simulink model "styremodell"  (R2023b)
settings: Solver=VariableStepAuto  StartTime=0.0  StopTime=30  RelTol=1e-3
undefined symbols (not defined in the file): areal_front, areal_side, areal_topp, bidrag_gir_front, bidrag_gir_side, bidrag_rull_side, bidrag_rull_topp, bidrag_stamp_front, bidrag_stamp_topp, Cd_front, Cd_side, Cd_topp, Fb, g, masse, r_Fb, r_motor_gir, r_motor_rull, r_motor_stamp, tetthet_vann, theta_motor_gir, theta_motor_rull, theta_motor_stamp, treghetsmoment_gir, treghetsmoment_rull, treghetsmoment_stamp
libraries: simulink_extras x8
settings Model: Creator=kristianbirkeland  LastModifiedBy=bmm1
settings DebuggingCC: UnconnectedInputMsg=warning  UnconnectedOutputMsg=warning  UnconnectedLineMsg=warning
settings ModelReferenceCC: EnableRefExpFcnMdlSchedulingChecks=on
settings RTWCC: DLArmComputeVersion=19.05

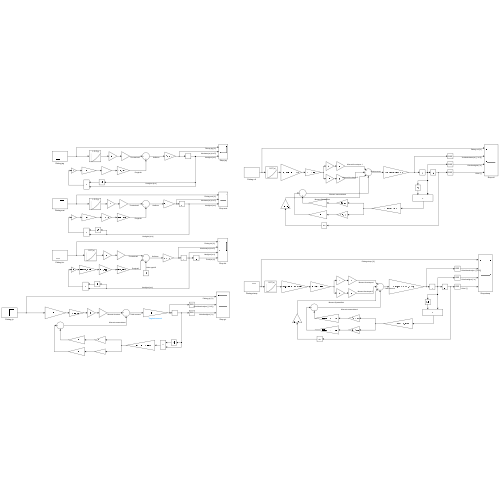
[thumbnail: Simulink's stored preview of the top-level diagram]
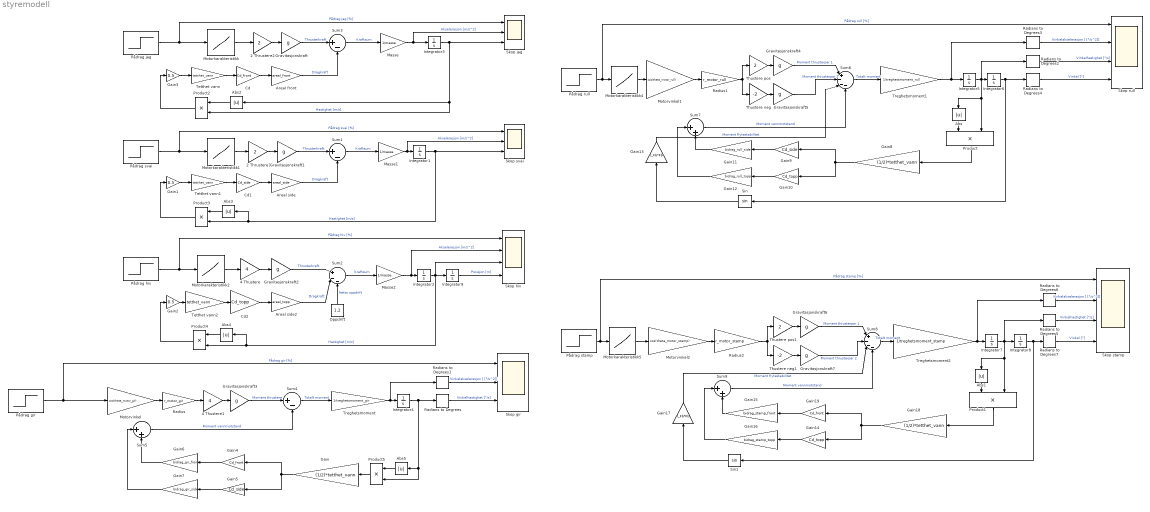
== system styremodell ==
  2 Thrustere1 : Gain  Gain=2
  2 Thrustere2 : Gain  Gain=2
  4 Thustere : Gain  Gain=4
  4 Thustere1 : Gain  Gain=4
  Abs{,1..5} (6 alike) : Abs  SaturateOnIntegerOverflow=off
  Areal front : Gain  Gain=areal_front
  Areal side : Gain  Gain=areal_side
  Areal side2 : Gain  Gain=areal_topp
  Cd : Gain  Gain=Cd_front
  Cd1 : Gain  Gain=Cd_side
  Cd2 : Gain  Gain=Cd_topp
  Gain : Gain  Gain=(1/2)*tetthet_vann
  Gain1 : Gain  Gain=0.5
  Gain10 : Gain  Gain=Cd_topp
  Gain11 : Gain  Gain=bidrag_rull_side
  Gain12 : Gain  Gain=bidrag_rull_topp
  Gain13 : Gain  Gain=r_Fb*Fb
  Gain14 : Gain  Gain=Cd_topp
  Gain15 : Gain  Gain=bidrag_stamp_front
  Gain16 : Gain  Gain=bidrag_stamp_topp
  Gain17 : Gain  Gain=r_Fb*Fb
  Gain18 : Gain  Gain=(1/2)*tetthet_vann
  Gain19 : Gain  Gain=Cd_front
  Gain2 : Gain  Gain=0.5
  Gain3 : Gain  Gain=0.5
  Gain4 : Gain  Gain=Cd_front
  Gain5 : Gain  Gain=Cd_side
  Gain6 : Gain  Gain=bidrag_gir_front
  Gain7 : Gain  Gain=bidrag_gir_side
  Gain8 : Gain  Gain=(1/2)*tetthet_vann
  Gain9 : Gain  Gain=Cd_side
  Gravitasjonskraft{,1..7} (8 alike) : Gain  Gain=g
  Integrator{1..5,7} (6 alike) : Integrator
  Integrator6 : Integrator  InitialCondition=pi/4
  Integrator8 : Integrator  InitialCondition=pi/4
  Integrator9 : Integrator  InitialCondition=1
  Masse : Gain  Gain=1/masse
  Masse1 : Gain  Gain=1/masse
  Masse2 : Gain  Gain=1/masse
  Motorkarakteristikk{,1..2,4..5} (5 alike) : Lookup_n-D  NumberOfTableDimensions=1  BreakpointsForDimension1="[0   12.5000   25.0000   37.5000   50.0000   62.5000   75.0000   87.5000  100.0000]"  Table="[0    0.0370    0.2589    0.5675    0.8927    1.2590    1.7264    2.2152    2.7880]"  InternalRulePriority=Speed  RndMeth=Simplest
  Motorvinkel : Gain  Gain=cos(theta_motor_gir)
  Motorvinkel1 : Gain  Gain=cos(theta_motor_rull)
  Motorvinkel2 : Gain  Gain=cos(theta_motor_stamp)
  Oppdrift : Constant  Value=1.2
  Product{,1..5} (6 alike) : Product
  Pådrag gir : Step  Time=0.5  After=0  SampleTime=0
  Pådrag hiv : Step  Time=3  After=100  SampleTime=0
  Pådrag jag : Step  Time=0.5  After=100  SampleTime=0
  Pådrag rull : Step  Time=10  After=28  SampleTime=0
  Pådrag stamp : Step  Time=10  After=31  SampleTime=0
  Pådrag svai : Step  Time=0.5  After=100  SampleTime=0
  Radians to Degrees{,1..7} (8 alike) : simulink_extras/Transformations/Radians to Degrees
  Radius : Gain  Gain=r_motor_gir
  Radius1 : Gain  Gain=r_motor_rull
  Radius2 : Gain  Gain=r_motor_stamp
  Sin : Trigonometry
  Sin1 : Trigonometry
  Skop gir : Scope  NumInputPorts=3
  Skop hiv : Scope  NumInputPorts=4
  Skop jag : Scope  NumInputPorts=3
  Skop rull : Scope  NumInputPorts=4
  Skop stamp : Scope  NumInputPorts=4
  Skop svai : Scope  NumInputPorts=3
  Sum1 : Sum  Inputs=|+-
  Sum2 : Sum  Inputs=|+--
  Sum3 : Sum  Inputs=|+-
  Sum4 : Sum  Inputs=|+-
  Sum5 : Sum  Inputs=|++
  Sum6 : Sum  Inputs=|+---
  Sum7 : Sum  Inputs=|++
  Sum8 : Sum  Inputs=|+---
  Sum9 : Sum  Inputs=|++
  Tetthet vann : Gain  Gain=tetthet_vann
  Tetthet vann1 : Gain  Gain=tetthet_vann
  Tetthet vann2 : Gain  Gain=tetthet_vann
  Thustere neg : Gain  Gain=-2
  Thustere neg1 : Gain  Gain=-2
  Thustere pos : Gain  Gain=2
  Thustere pos1 : Gain  Gain=2
  Treghetsmoment : Gain  Gain=1/treghetsmoment_gir
  Treghetsmoment1 : Gain  Gain=1/treghetsmoment_rull
  Treghetsmoment2 : Gain  Gain=1/treghetsmoment_stamp
  wires:
  Gravitasjonskraft1/1 -> Sum1/1  "Thrusterkraft"
  2 Thrustere1/1 -> Gravitasjonskraft1/1
  Sum1/1 -> Masse1/1  "Kraftsum"
  Gain1/1 -> Tetthet vann1/1
  Tetthet vann1/1 -> Cd1/1
  Pådrag svai/1 -> Skop svai/1, Motorkarakteristikk1/1  "Pådrag svai [%]"
  Masse1/1 -> Skop svai/2, Integrator1/1  "Akselerasjon [m/s^2]"
  Cd1/1 -> Areal side/1
  Integrator1/1 -> Abs3/1, Product3/2, Skop svai/3  "Hastighet [m/s]"
  Motorkarakteristikk1/1 -> 2 Thrustere1/1
  Areal side/1 -> Sum1/2  "Dragkraft"
  Product3/1 -> Gain1/1
  Integrator3/1 -> Product2/2, Abs2/1, Skop jag/3  "Hastighet [m/s]"
  Motorkarakteristikk/1 -> 2 Thrustere2/1
  Pådrag jag/1 -> Skop jag/1, Motorkarakteristikk/1  "Pådrag jag [%]"
  Cd/1 -> Areal front/1
  Masse/1 -> Skop jag/2, Integrator3/1  "Akselerasjon [m/s^2]"
  Areal front/1 -> Sum3/2  "Dragkraft"
  Product2/1 -> Gain3/1
  2 Thrustere2/1 -> Gravitasjonskraft/1
  Gravitasjonskraft/1 -> Sum3/1  "Thrusterkraft"
  Sum3/1 -> Masse/1  "Kraftsum"
  Gain3/1 -> Tetthet vann/1
  Tetthet vann/1 -> Cd/1
  Motorkarakteristikk2/1 -> 4 Thustere/1
  Pådrag hiv/1 -> Skop hiv/1, Motorkarakteristikk2/1  "Pådrag hiv [%]"
  Cd2/1 -> Areal side2/1
  Masse2/1 -> Skop hiv/2, Integrator2/1  "Akselerasjon [m/s^2]"
  Areal side2/1 -> Sum2/2  "Dragkraft"
  4 Thustere/1 -> Gravitasjonskraft2/1
  Gravitasjonskraft2/1 -> Sum2/1  "Thrusterkraft"
  Sum2/1 -> Masse2/1  "Kraftsum"
  Gain2/1 -> Tetthet vann2/1
  Tetthet vann2/1 -> Cd2/1
  Oppdrift/1 -> Sum2/3  "Netto oppdrift"
  Sum4/1 -> Treghetsmoment/1  "Totalt moment"
  4 Thustere1/1 -> Gravitasjonskraft3/1
  Treghetsmoment/1 -> Radians to Degrees1/1, Integrator4/1
  Gravitasjonskraft3/1 -> Sum4/1  "Moment thrustere"
  Integrator4/1 -> Abs5/1, Product5/2, Radians to Degrees/1
  Pådrag gir/1 -> Motorvinkel/1, Skop gir/1  "Pådrag gir [%]"
  Motorvinkel/1 -> Radius/1
  Radius/1 -> 4 Thustere1/1
  Gain/1 -> Gain5/1, Gain4/1
  Product5/1 -> Gain/1
  Gain4/1 -> Gain6/1
  Gain5/1 -> Gain7/1
  Gain7/1 -> Sum5/1
  Gain6/1 -> Sum5/2
  Sum5/1 -> Sum4/2  "Moment vannmotstand"
  Radians to Degrees/1 -> Skop gir/3  "Vinkelhastighet [°/s]"
  Radians to Degrees1/1 -> Skop gir/2  "Vinkelakselerasjon [ [°/s^2]]"
  Radius1/1 -> Thustere neg/1, Thustere pos/1
  Gain9/1 -> Gain11/1
  Pådrag rull/1 -> Motorkarakteristikk4/1, Skop rull/1  "Pådrag rull [%]"
  Gain12/1 -> Sum7/1
  Gain8/1 -> Gain10/1, Gain9/1
  Gravitasjonskraft4/1 -> Sum6/1  "Moment thrusterpar 1"
  Gain11/1 -> Sum7/2
  Treghetsmoment1/1 -> Radians to Degrees3/1, Integrator5/1
  Motorvinkel1/1 -> Radius1/1
  Radians to Degrees2/1 -> Skop rull/3  "Vinkelhastighet [°/s]"
  Integrator5/1 -> Abs/1, Product/2, Integrator6/1, Radians to Degrees2/1
  Motorkarakteristikk4/1 -> Motorvinkel1/1
  Product/1 -> Gain8/1
  Gain10/1 -> Gain12/1
  Radians to Degrees3/1 -> Skop rull/2  "Vinkelakselerasjon [ [°/s^2]]"
  Sum6/1 -> Treghetsmoment1/1  "Totalt moment"
  Thustere pos/1 -> Gravitasjonskraft4/1
  Thustere neg/1 -> Gravitasjonskraft5/1
  Gravitasjonskraft5/1 -> Sum6/2  "Moment thrusterpar 2"
  Radians to Degrees4/1 -> Skop rull/4  "Vinkel [°]"
  Sum7/1 -> Sum6/4  "Moment vannmotstand"
  Integrator6/1 -> Sin/1, Radians to Degrees4/1
  Gain13/1 -> Sum6/3  "Moment flytestabilitet"
  Sin/1 -> Gain13/1
  Abs/1 -> Product/1
  Pådrag stamp/1 -> Skop stamp/1, Motorkarakteristikk5/1  "Pådrag stamp [%]"
  Motorkarakteristikk5/1 -> Motorvinkel2/1
  Gain16/1 -> Sum9/1
  Gain19/1 -> Gain15/1
  Thustere neg1/1 -> Gravitasjonskraft7/1
  Gain18/1 -> Gain14/1, Gain19/1
  Thustere pos1/1 -> Gravitasjonskraft6/1
  Motorvinkel2/1 -> Radius2/1
  Sum9/1 -> Sum8/4  "Moment vannmotstand"
  Radians to Degrees5/1 -> Skop stamp/3  "Vinkelhastighet [°/s]"
  Gravitasjonskraft7/1 -> Sum8/2  "Moment thrusterpar 2"
  Abs1/1 -> Product1/1
  Radians to Degrees6/1 -> Skop stamp/2  "Vinkelakselerasjon [ [°/s^2]]"
  Radians to Degrees7/1 -> Skop stamp/4  "Vinkel [°]"
  Treghetsmoment2/1 -> Radians to Degrees6/1, Integrator7/1
  Gain15/1 -> Sum9/2
  Radius2/1 -> Thustere pos1/1, Thustere neg1/1
  Gravitasjonskraft6/1 -> Sum8/1  "Moment thrusterpar 1"
  Gain17/1 -> Sum8/3  "Moment flytestabilitet"
  Gain14/1 -> Gain16/1
  Integrator7/1 -> Radians to Degrees5/1, Abs1/1, Product1/2, Integrator8/1
  Sum8/1 -> Treghetsmoment2/1  "Totalt moment"
  Sin1/1 -> Gain17/1
  Integrator8/1 -> Sin1/1, Radians to Degrees7/1
  Product1/1 -> Gain18/1
  Integrator9/1 -> Skop hiv/4  "Posisjon [m]"
  Abs2/1 -> Product2/1
  Abs3/1 -> Product3/1
  Integrator2/1 -> Abs4/1, Product4/2, Integrator9/1, Skop hiv/3  "Hastighet [m/s]"
  Abs4/1 -> Product4/1
  Product4/1 -> Gain2/1
  Abs5/1 -> Product5/1
